simulink model "pedal"  (Simulink 3.00)
settings: Solver=ode45  StartTime=0.0  StopTime=10.0  RelTol=1e-3
values from neighbouring files (symbols this model uses):
  x10 = 0    [v515.m]    (also in v516.m; v517.m)
  x20 = 0    [v515.m]    (also in v516.m; v517.m)
settings Model: LastModifiedBy=Administrator

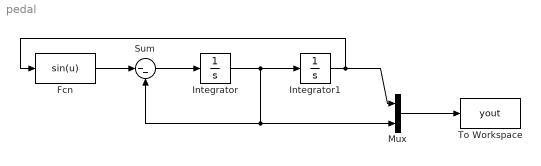
== system pedal ==
  Fcn : Fcn  Expr=sin(u)
  Integrator : Integrator  ExternalReset=none  InitialConditionSource=internal  InitialCondition=x20  LimitOutput=off  UpperSaturationLimit=inf  LowerSaturationLimit=-inf  ShowSaturationPort=off  ShowStatePort=off  AbsoluteTolerance=auto
  Integrator1 : Integrator  ExternalReset=none  InitialConditionSource=internal  InitialCondition=x10  LimitOutput=off  UpperSaturationLimit=inf  LowerSaturationLimit=-inf  ShowSaturationPort=off  ShowStatePort=off  AbsoluteTolerance=auto
  Mux : Mux  Inputs=2
  Sum : Sum  Inputs=|--  SaturateOnIntegerOverflow=on
  To Workspace : ToWorkspace  VariableName=yout  SampleTime=-1  SaveFormat=Matrix
  wires:
  Fcn/1 -> Sum/1
  Sum/1 -> Integrator/1
  Integrator/1 -> Integrator1/1, Mux/2, Sum/2
  Integrator1/1 -> Mux/1, Fcn/1
  Mux/1 -> To Workspace/1
